simulink model "sxema"  (R2018b)
settings: Solver=VariableStepAuto  StartTime=0.0  StopTime=100  MaxStep=0.01  RelTol=1e-3
undefined symbols (not defined in the file or in its folder): K
settings Model: Creator=kekos  LastModifiedBy=kekos

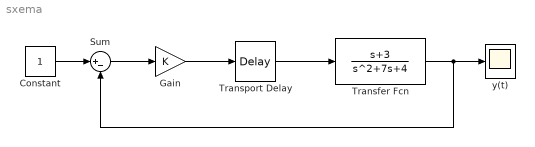
== system sxema ==
  Constant : Constant
  Gain : Gain  Gain=K
  Sum : Sum  Inputs=|+-
  Transfer Fcn : TransferFcn  Numerator=[1 3]  Denominator=[1 7 4]
  Transport Delay : TransportDelay  DelayTime=10
  y(t) : Scope
  wires:
  Gain/1 -> Transport Delay/1
  Sum/1 -> Gain/1
  Constant/1 -> Sum/1
  Transport Delay/1 -> Transfer Fcn/1
  Transfer Fcn/1 -> y(t)/1, Sum/2
